simulink model "cascade_realization"  (R2020b)
settings: Solver=VariableStepAuto  StartTime=0.0  StopTime=10.0  RelTol=1e-3
settings Model: Creator=shubham sharma  LastModifiedBy=shubham sharma

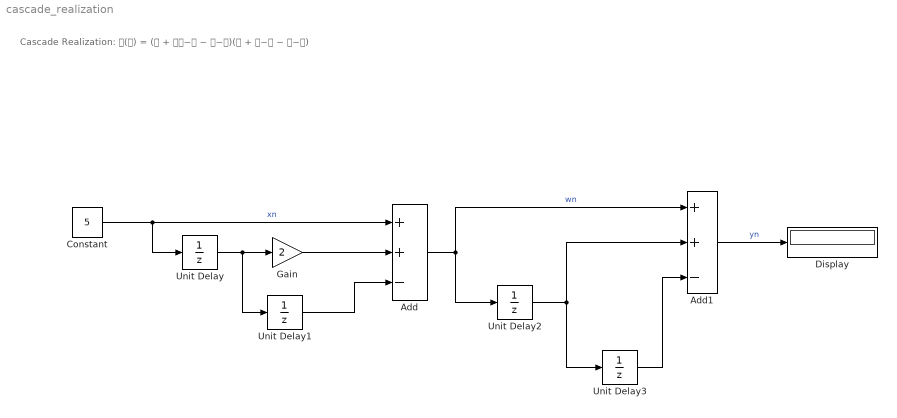
== system cascade_realization ==
  note: Cascade Realization:
      | 𝐇(𝐳) = (𝟏 + 𝟐𝐳−𝟏 − 𝐳−𝟐)(𝟏 + 𝐳−𝟏 − 𝐳−𝟐)
  Add : Sum  Inputs=++-
  Add1 : Sum  Inputs=++-
  Constant : Constant  Value=5
  Display : Display
  Gain : Gain  Gain=2
  Unit Delay{,1..3} (4 alike) : UnitDelay  SampleTime=-1  HasFrameUpgradeWarning=on
  wires:
  Constant/1 -> Unit Delay/1, Add/1  "xn"
  Gain/1 -> Add/2
  Unit Delay/1 -> Unit Delay1/1, Gain/1
  Unit Delay1/1 -> Add/3
  Add/1 -> Unit Delay2/1, Add1/1  "wn"
  Unit Delay2/1 -> Unit Delay3/1, Add1/2
  Unit Delay3/1 -> Add1/3
  Add1/1 -> Display/1  "yn"
